simulink model "reg_model"  (R2024a)
settings: Solver=FixedStepAuto  StartTime=0.0  StopTime=10  FixedStep=0.0001  MinStep=1e-8  RelTol=1e-8  AbsTol=1e-8
model workspace (MAT data in the model file):
  A = [11  -2  13; 6  -1  6; -6  -1  -8]
  B = [2; 0; 0]
  K = [-4 2.4167 -3]
values from neighbouring files (symbols this model uses):
  K1_full_standard = K1_full*T^(-1)    [reg.m]
  K2_full_standard = K2_full*T^(-1)    [reg.m]
  K3_full_standard = K3_full*T^(-1)    [reg.m]
settings Model: Creator=ventus  LastModifiedBy=ventus

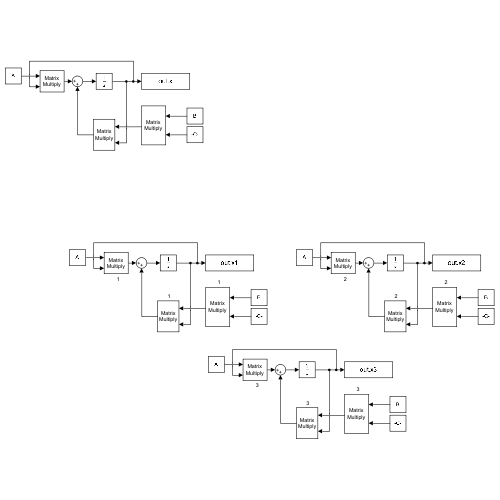
[thumbnail: Simulink's stored preview of the top-level diagram]
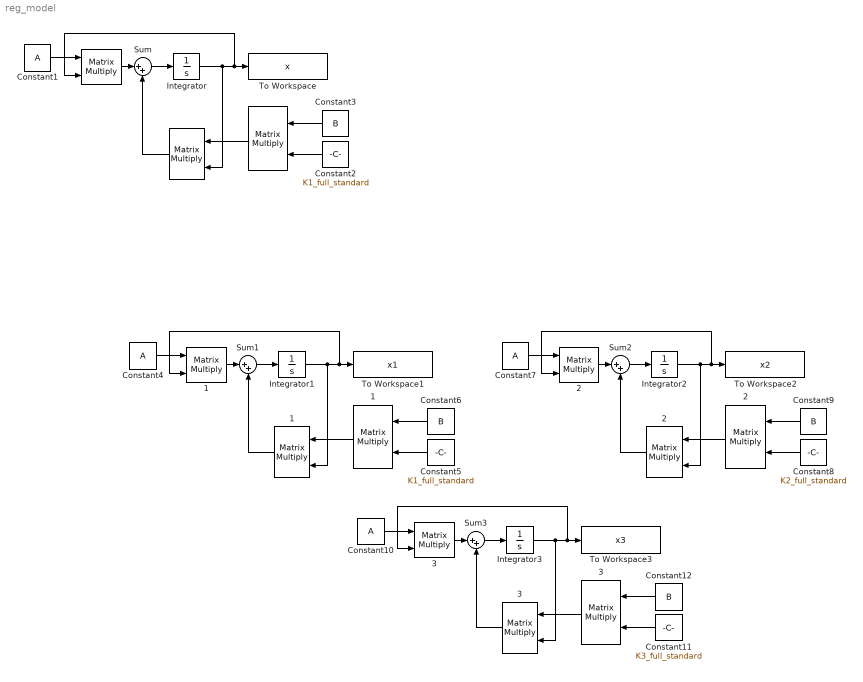
== system reg_model ==
   {,1..3} (4 alike) : Product  Multiplication=Matrix(*)
    {,1..3} (4 alike) : Product  Multiplication=Matrix(*)
     {,1..3} (4 alike) : Product  Multiplication=Matrix(*)
  Constant{1,4,7,10} (4 alike) : Constant  Value=A  VectorParams1D=off
  Constant11 : Constant  Value=K3_full_standard  VectorParams1D=off
  Constant{3,6,9,12} (4 alike) : Constant  Value=B  VectorParams1D=off
  Constant2 : Constant  Value=K1_full_standard  VectorParams1D=off
  Constant5 : Constant  Value=K1_full_standard  VectorParams1D=off
  Constant8 : Constant  Value=K2_full_standard  VectorParams1D=off
  Integrator{,1..3} (4 alike) : Integrator  InitialCondition=[1; 1; 1]
  Sum{,1..3} (4 alike) : Sum  Inputs=|++
  To Workspace : ToWorkspace  VariableName=x  SaveFormat=Timeseries  SampleTime=-1
  To Workspace1 : ToWorkspace  VariableName=x1  SaveFormat=Timeseries  SampleTime=-1
  To Workspace2 : ToWorkspace  VariableName=x2  SaveFormat=Timeseries  SampleTime=-1
  To Workspace3 : ToWorkspace  VariableName=x3  SaveFormat=Timeseries  SampleTime=-1
  wires:
  Integrator/1 -> To Workspace/1, "   "/2, " "/2
  Constant2/1 -> "  "/2
  "  "/1 -> " "/1
  " "/1 -> Sum/2
  Sum/1 -> Integrator/1
  Constant3/1 -> "  "/1
  Constant1/1 -> "   "/1
  "   "/1 -> Sum/1
  " 1"/1 -> Sum1/2
  Constant6/1 -> "  1"/1
  "  1"/1 -> " 1"/1
  "   1"/1 -> Sum1/1
  Sum1/1 -> Integrator1/1
  Constant4/1 -> "   1"/1
  Constant5/1 -> "  1"/2
  Integrator1/1 -> To Workspace1/1, "   1"/2, " 1"/2
  " 2"/1 -> Sum2/2
  Constant9/1 -> "  2"/1
  "  2"/1 -> " 2"/1
  "   2"/1 -> Sum2/1
  Sum2/1 -> Integrator2/1
  Constant7/1 -> "   2"/1
  Constant8/1 -> "  2"/2
  Integrator2/1 -> To Workspace2/1, "   2"/2, " 2"/2
  " 3"/1 -> Sum3/2
  Constant12/1 -> "  3"/1
  "  3"/1 -> " 3"/1
  "   3"/1 -> Sum3/1
  Sum3/1 -> Integrator3/1
  Constant10/1 -> "   3"/1
  Constant11/1 -> "  3"/2
  Integrator3/1 -> To Workspace3/1, "   3"/2, " 3"/2
